simulink model "swarch"  (R2022b)
settings: Solver=VariableStepAuto  StartTime=0.0  StopTime=10.0  RelTol=1e-3
libraries: SignalEditorBlockLib x1
settings Model: Creator=alber  LastModifiedBy=alber

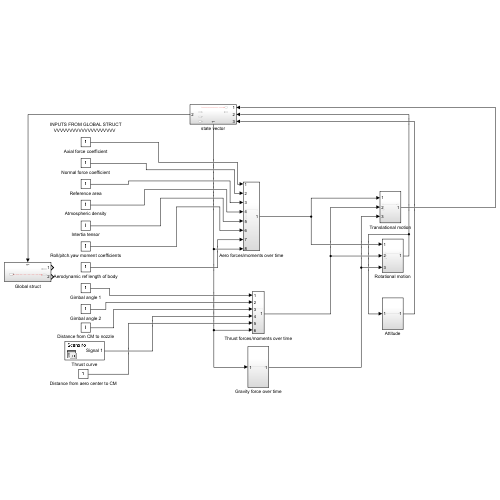
[thumbnail: Simulink's stored preview of the top-level diagram]
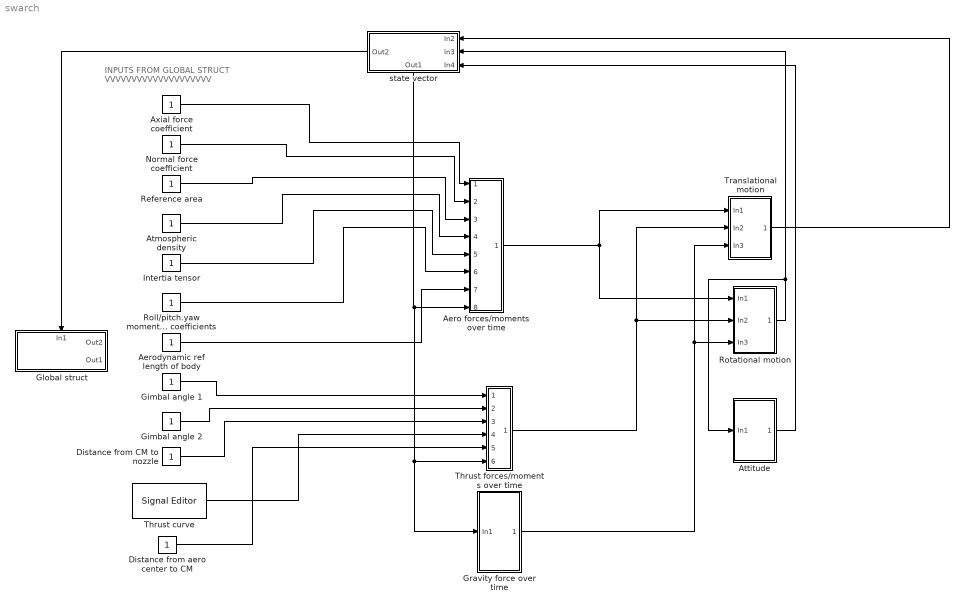
== system swarch ==
  note: INPUTS FROM GLOBAL STRUCT
      |    VVVVVVVVVVVVVVVVVVVV
  Aero forces/moments over time : Subsystem
  Aerodynamic ref length of body : Constant
  Atmospheric density : Constant
  Attitude : Subsystem
  Axial force coefficient : Constant
  Distance from CM to nozzle : Constant
  Distance from aero center to CM : Constant
  Gimbal angle 1 : Constant
  Gimbal angle 2 : Constant
  Global struct : Subsystem
      settings: PortSchema="{\"entries\":[{\"content\":{\"sides\":[{\"content\":{\"connectorIds\":[]},\"type\":\"ConnectorPlacement.EquallySpacedRectSide\",\"uuid\":\"dc63b528-eddd-4be5-8fca-bfbd7a0c5e3b\"},{\"content\":{\"connectorIds\":[\"Out1\",\"Out2\"],\"side\":\"RIGHT\"},\"type\":\"ConnectorPlacement.EquallySpacedRectSide\",\"uuid\":\"67969a92-87c7-47ef-8bff-b787d64f7abe\"},{\"content\":{\"connectorIds\":[\"In1\"],\"side\":\"TOP\"},\"type\":\"ConnectorPlacement.EquallySpacedRectSide\",\"uuid\":\"6f8a2e97-e29a-4bfb-b3a7-aa987b9cedf4\"}]},\"type\":\"ConnectorPlacement.EquallySpacedConnector\",\"uuid\":\"a05b6623-0bf9-41eb-9c2b-86a719edc676\"}],\"packageUris\":[\"http://schema.mathworks.com/mf0/Connector/R2020b\"],\"version\":\"1.0\"}"
  Gravity force over time : Subsystem
  Intertia tensor : Constant
  Normal force coefficient : Constant
  Reference area : Constant
  Roll/pitch.yaw moment coefficients : Constant
  Rotational motion : Subsystem
  Thrust curve : SignalEditorBlockLib/Signal Editor  FileName=untitled.mat  ActiveScenario=Scenario  ActiveSignal=Signal 1  IsBus=off  OutputBusObjectStr=Bus: BusObject  SampleTime=0  Interpolate=off  ZeroCross=off  OutputAfterFinalValue=Setting to zero  Unit=inherit  PreserveSignalName=on
  Thrust forces/moments over time : Subsystem
  Translational motion : Subsystem
  state vector : Subsystem
      settings: PortSchema="{\"entries\":[{\"content\":{\"sides\":[{\"content\":{\"connectorIds\":[\"Out2\"]},\"type\":\"ConnectorPlacement.EquallySpacedRectSide\",\"uuid\":\"979422d1-faef-4f5a-abaa-036a676295a0\"},{\"content\":{\"connectorIds\":[\"In1\",\"In2\",\"In3\"],\"side\":\"RIGHT\"},\"type\":\"ConnectorPlacement.EquallySpacedRectSide\",\"uuid\":\"de691626-f81b-43c5-9177-3c2e0ae3af99\"},{\"content\":{\"connectorIds\":[],\"side\":\"TOP\"},\"type\":\"ConnectorPlacement.EquallySpacedRectSide\",\"uuid\":\"4c307ef1-2e7e-47db-9a54-bc8d79521762\"},{\"content\":{\"connectorIds\":[\"Out1\"],\"side\":\"BOTTOM\"},\"type\":\"ConnectorPlacement.EquallySpacedRectSide\",\"uuid\":\"636d924a-2936-4014-9335-2ebc508efd80\"}]},\"type\":\"ConnectorPlacement.EquallySpacedConnector\",\"uuid\":\"b6df6972-c27b-4f76-bbbc-c80fecdbc406\"}],\"packageUris\":[\"http://schema.mathworks.com/mf0/Connector/R2020b\"],\"version\":\"1.0\"}"
  wires:
  Aero forces/moments over time/1(Out1) -> Translational motion/1(In1), Rotational motion/1(In1)
  Thrust forces/moments over time/1(Out1) -> Translational motion/2(In2), Rotational motion/2(In2)
  Gravity force over time/1(Out1) -> Translational motion/3(In3), Rotational motion/3(In3)
  Axial force coefficient/1 -> Aero forces/moments over time/1(In1)
  Normal force coefficient/1 -> Aero forces/moments over time/2(In2)
  Reference area/1 -> Aero forces/moments over time/3(In3)
  Atmospheric density/1 -> Aero forces/moments over time/4(In4)
  Gimbal angle 1/1 -> Thrust forces/moments over time/1(In1)
  Gimbal angle 2/1 -> Thrust forces/moments over time/2(In2)
  Distance from CM to nozzle/1 -> Thrust forces/moments over time/3(In3)
  Thrust curve/1 -> Thrust forces/moments over time/4(In4)
  Distance from aero center to CM/1 -> Thrust forces/moments over time/5(In5)
  state vector/1(Out1) -> Aero forces/moments over time/8(In5), Gravity force over time/1(In1), Thrust forces/moments over time/6(In6)
  Translational motion/1(Out1) -> state vector/1(In2)
  Rotational motion/1(Out1) -> Attitude/1(In1), state vector/2(In3)
  Attitude/1(Out1) -> state vector/3(In4)
  state vector/2(Out2) -> Global struct/1(In1)
  Intertia tensor/1 -> Aero forces/moments over time/5(In6)
  Roll/pitch.yaw moment coefficients/1 -> Aero forces/moments over time/6(In7)
  Aerodynamic ref length of body/1 -> Aero forces/moments over time/7(In8)

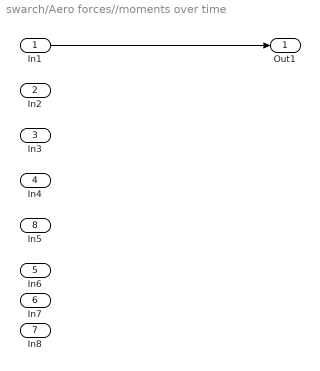
== system swarch/Aero forces//moments over time ==
  In1 : Inport
  In2 : Inport  Port=2
  In3 : Inport  Port=3
  In4 : Inport  Port=4
  In6 : Inport  Port=5
  In7 : Inport  Port=6
  In8 : Inport  Port=7
  In5 : Inport  Port=8
  Out1 : Outport
  wires:
  In1/1 -> Out1/1

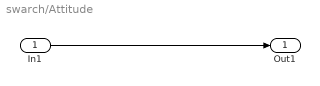
== system swarch/Attitude ==
  In1 : Inport
  Out1 : Outport
  wires:
  In1/1 -> Out1/1

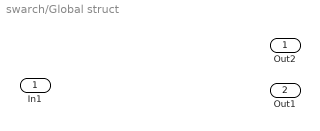
== system swarch/Global struct ==
  In1 : Inport
  Out2 : Outport
  Out1 : Outport  Port=2
  wires:
  ? -> Out1/1

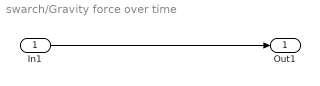
== system swarch/Gravity force over time ==
  In1 : Inport
  Out1 : Outport
  wires:
  In1/1 -> Out1/1

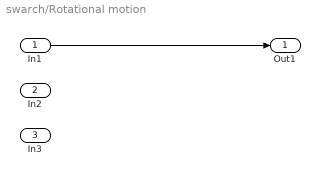
== system swarch/Rotational motion ==
  In1 : Inport
  In2 : Inport  Port=2
  In3 : Inport  Port=3
  Out1 : Outport
  wires:
  In1/1 -> Out1/1

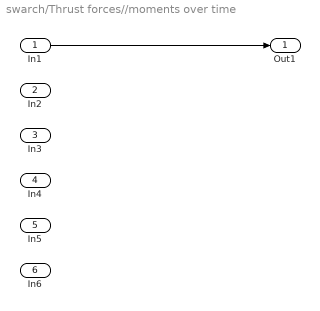
== system swarch/Thrust forces//moments over time ==
  In1 : Inport
  In2 : Inport  Port=2
  In3 : Inport  Port=3
  In4 : Inport  Port=4
  In5 : Inport  Port=5
  In6 : Inport  Port=6
  Out1 : Outport
  wires:
  In1/1 -> Out1/1

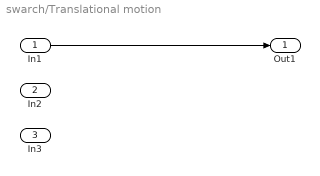
== system swarch/Translational motion ==
  In1 : Inport
  In2 : Inport  Port=2
  In3 : Inport  Port=3
  Out1 : Outport
  wires:
  In1/1 -> Out1/1

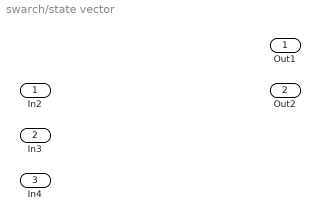
== system swarch/state vector ==
  In2 : Inport
  In3 : Inport  Port=2
  In4 : Inport  Port=3
  Out1 : Outport
  Out2 : Outport  Port=2
  wires:
  ? -> Out1/1
